simulink library "TestLib_BCM_Manager"  (Simulink 7.5)
settings: Solver=ode1  StartTime=0.0  StopTime=Inf  FixedStep=0.001  RelTol=1e-3
PostLoadFcn:
  | , if any(exist('dsrtsu_mdlpostloadfcn', 'file') == [2, 3, 6]), try dsrtsu_mdlpostloadfcn('Execute', bdroot); catch fprintf('Error in PostLoadFcn (dsrtsu_mdlpostloadfcn) for model "%s":\n %s\n', bdroot, lasterr); end, end,
undefined symbols (not defined in the file): cal, tloop
libraries: simulink x92, EC2_libraries x74
(part 2 of 2)

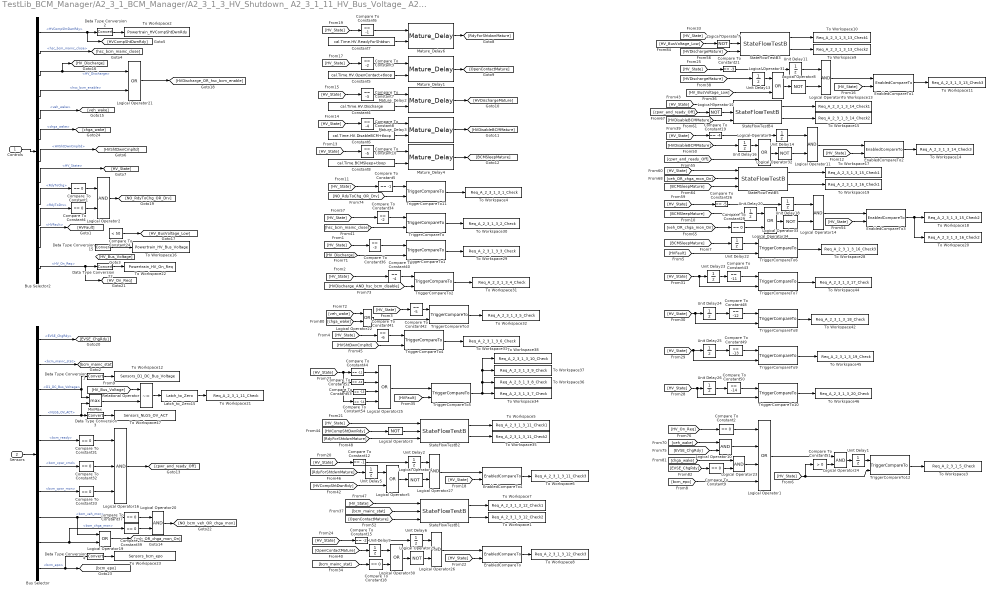
== system TestLib_BCM_Manager/A2_3_1_BCM_Manager/A2_3_1_3_HV_Shutdown_ A2_3_1_11_HV_Bus_Voltage_ A2_3_1_5_Startup_to_Shutdown ==
  Controls : Inport  OutDataType=fixdt(1, 16)  OutScaling=2^0
  Sensors : Inport  Port=2  OutDataType=fixdt(1, 16)  OutScaling=2^0
  Bus Selector : BusSelector  OutputSignals=Analog.EVSE_ChgRdy,Sensors_CAN.BCM_HS_Tx.BCM_Status.bcm_mainc_stat,Sensors_CAN.MCU_HS_Tx.M167_Voltage_Info.D1_DC_Bus_Voltage,Sensors_CAN.OBC_HS_Tx.NLG5_ACT_I.NLG5_OV_ACT,Sensors_CAN.BCM_HS_Tx.BCM_Status.bcm_ready,Sensors_CAN.BCM_HS_Tx.BCM_Status.bcm_cpwr_cmd,Sensors_CAN.BCM_HS_Tx.BCM_Status.bcm_cpwr_mon,Sensors_CAN.BCM_HS_Tx.BCM_Data1.bcm_veh_mon,Sensors_CAN.BCM_HS_Tx.BCM_Data1.bcm_chga_mon,Sensors_CAN.BCM_HS_Tx.BCM_Status.bcm_epo
  Bus Selector2 : BusSelector  OutputSignals=Powertrain_SC_Controls.HV_Status.HVCompShtDwnRdy,Powertrain_SC_Controls.BCM_Control.hsc_bcm_mainc_close,Powertrain_SC_Controls.HV_Status.HV_Discharge,Powertrain_SC_Controls.BCM_Control.hsc_bcm_enable,Powertrain_SC_Controls.BCM_Control.veh_wake,Powertrain_SC_Controls.BCM_Control.chga_wake,Powertrain_SC_Controls.HV_Status.HVShtDwnCmpltd,Powertrain_SC_Controls.HV_Status.HV_State,Powertrain_SC_Controls.HV_Status.RdyToChg,Powertrain_SC_Controls.HV_Status.RdyToDrv,Powertrain_SC_Controls.HV_Status.HVFault,Powertrain_SC_Controls.HV_Status.HV_On_Req
  Compare To Constant{1..2,4,9,18,29,31..33,37,39} (11 alike) : simulink/Logic and Bit Operations/Compare To Constant  SystemSampleTime=-1  relop===  const=0  LogicOutDataTypeMode=uint8
  Compare To Constant10 : simulink/Logic and Bit Operations/Compare To Constant  SystemSampleTime=-1  relop===  const=-5  LogicOutDataTypeMode=uint8
  Compare To Constant12 : simulink/Logic and Bit Operations/Compare To Constant  SystemSampleTime=-1  relop===  const=-1  LogicOutDataTypeMode=uint8
  Compare To Constant15 : simulink/Logic and Bit Operations/Compare To Constant  SystemSampleTime=-1  relop===  const=-2  LogicOutDataTypeMode=uint8
  Compare To Constant19 : simulink/Logic and Bit Operations/Compare To Constant  SystemSampleTime=-1  relop===  const=-4  LogicOutDataTypeMode=uint8
  Compare To Constant21 : simulink/Logic and Bit Operations/Compare To Constant  SystemSampleTime=-1  relop===  const=-3  LogicOutDataTypeMode=uint8
  Compare To Constant24 : simulink/Logic and Bit Operations/Compare To Constant  SystemSampleTime=-1  relop=<  const=50  LogicOutDataTypeMode=boolean
  Compare To Constant26 : simulink/Logic and Bit Operations/Compare To Constant  SystemSampleTime=-1  relop===  const=-5  LogicOutDataTypeMode=uint8
  Compare To Constant3 : simulink/Logic and Bit Operations/Compare To Constant  SystemSampleTime=-1  relop===  const=-2  LogicOutDataTypeMode=uint8
  Compare To Constant34 : simulink/Logic and Bit Operations/Compare To Constant  SystemSampleTime=-1  relop===  const=-2  LogicOutDataTypeMode=uint8
  Compare To Constant36 : simulink/Logic and Bit Operations/Compare To Constant  SystemSampleTime=-1  relop===  const=-3  LogicOutDataTypeMode=uint8
  Compare To Constant40 : simulink/Logic and Bit Operations/Compare To Constant  SystemSampleTime=-1  relop===  const=-4  LogicOutDataTypeMode=uint8
  Compare To Constant41 : simulink/Logic and Bit Operations/Compare To Constant  SystemSampleTime=-1  relop===  const=-6  LogicOutDataTypeMode=uint8
  Compare To Constant42 : simulink/Logic and Bit Operations/Compare To Constant  SystemSampleTime=-1  relop===  const=-5  LogicOutDataTypeMode=uint8
  Compare To Constant43 : simulink/Logic and Bit Operations/Compare To Constant  SystemSampleTime=-1  relop===  const=-11  LogicOutDataTypeMode=uint8
  Compare To Constant44 : simulink/Logic and Bit Operations/Compare To Constant  SystemSampleTime=-1  relop===  const=-11  LogicOutDataTypeMode=uint8
  Compare To Constant48 : simulink/Logic and Bit Operations/Compare To Constant  SystemSampleTime=-1  relop===  const=-12  LogicOutDataTypeMode=uint8
  Compare To Constant49 : simulink/Logic and Bit Operations/Compare To Constant  SystemSampleTime=-1  relop===  const=-13  LogicOutDataTypeMode=uint8
  Compare To Constant5 : simulink/Logic and Bit Operations/Compare To Constant  SystemSampleTime=-1  relop===  const=-1  LogicOutDataTypeMode=uint8
  Compare To Constant50 : simulink/Logic and Bit Operations/Compare To Constant  SystemSampleTime=-1  relop===  const=-14  LogicOutDataTypeMode=uint8
  Compare To Constant51 : simulink/Logic and Bit Operations/Compare To Constant  SystemSampleTime=-1  relop=>  const=0  LogicOutDataTypeMode=uint8
  Compare To Constant52 : simulink/Logic and Bit Operations/Compare To Constant  SystemSampleTime=-1  relop===  const=-12  LogicOutDataTypeMode=uint8
  Compare To Constant53 : simulink/Logic and Bit Operations/Compare To Constant  SystemSampleTime=-1  relop===  const=-13  LogicOutDataTypeMode=uint8
  Compare To Constant54 : simulink/Logic and Bit Operations/Compare To Constant  SystemSampleTime=-1  relop===  const=-14  LogicOutDataTypeMode=uint8
  Compare To Constant6 : simulink/Logic and Bit Operations/Compare To Constant  SystemSampleTime=-1  relop===  const=-1  LogicOutDataTypeMode=uint8
  Compare To Constant7 : simulink/Logic and Bit Operations/Compare To Constant  SystemSampleTime=-1  relop===  const=-3  LogicOutDataTypeMode=uint8
  Compare To Constant8 : simulink/Logic and Bit Operations/Compare To Constant  SystemSampleTime=-1  relop===  const=-4  LogicOutDataTypeMode=uint8
  Constant4 : Constant  Value=cal.Time.HV.Discharge  VectorParams1D=off
  Constant5 : Constant  Value=cal.Time.HV.OpenContact+tloop  VectorParams1D=off
  Constant6 : Constant  Value=cal.Time.HV.DisableBCM+tloop  VectorParams1D=off
  Constant7 : Constant  Value=cal.Time.HV.ReadyForShtdwn  VectorParams1D=off
  Constant8 : Constant  Value=cal.Time.BCMSleep+tloop  VectorParams1D=off
  Data Type Conversion{1..4,15,22} (6 alike) : DataTypeConversion  OutDataType=fixdt(1, 16)  OutScaling=2^0
  EnabledCompareTo : EC2_libraries/EnabledCompareTo  SystemSampleTime=-1  exp_val=-2
  EnabledCompareTo1 : EC2_libraries/EnabledCompareTo  SystemSampleTime=-1  exp_val=-3
  EnabledCompareTo2 : EC2_libraries/EnabledCompareTo  SystemSampleTime=-1  exp_val=-4
  EnabledCompareTo3 : EC2_libraries/EnabledCompareTo  SystemSampleTime=-1  exp_val=-5
  EnabledCompareTo4 : EC2_libraries/EnabledCompareTo  SystemSampleTime=-1  exp_val=-1
  Latch_to_Zero15 : EC2_libraries/Latch_to_Zero  SystemSampleTime=-1
  Logical Operator1 : Logic  Operator=OR  Inputs=4  AllPortsSameDT=off  OutDataTypeMode=boolean  OutDataTypeStr=boolean
  Logical Operator{2,6,10..11,14,20,23..24,26..27} (10 alike) : Logic  AllPortsSameDT=off  OutDataTypeMode=boolean  OutDataTypeStr=boolean
  Logical Operator{3..4,7..8,12,29,32..33} (8 alike) : Logic  Operator=NOT  AllPortsSameDT=off  OutDataTypeMode=boolean  OutDataTypeStr=boolean
  Logical Operator16 : Logic  Inputs=3  AllPortsSameDT=off  OutDataTypeMode=boolean  OutDataTypeStr=boolean
  Logical Operator{5,9,19,21..22,30..31,34} (8 alike) : Logic  Operator=OR  AllPortsSameDT=off  OutDataTypeMode=boolean  OutDataTypeStr=boolean
  Logical Operator25 : Logic  Operator=OR  Inputs=4  AllPortsSameDT=off  OutDataTypeMode=boolean  OutDataTypeStr=boolean
  Mature_Delay{1..4,6} (5 alike) : EC2_libraries/Mature_Delay  SystemSampleTime=-1
  MinMax : MinMax  Function=max  Inputs=2  OutDataType=fixdt(1, 16)  OutScaling=2^0
  Relational Operator : RelationalOperator  Operator=~=  LogicOutDataTypeMode=boolean  LogicDataType=fixdt(0, 8)  OutDataTypeStr=boolean
  StateFlowTestB1 : EC2_libraries/StateFlowTestB  SystemSampleTime=-1  StateBase=-2  PrimaryState=-3  SecondaryState=-12
  StateFlowTestB2 : EC2_libraries/StateFlowTestB  SystemSampleTime=-1  StateBase=-1  PrimaryState=-2  SecondaryState=-11
  StateFlowTestB3 : EC2_libraries/StateFlowTestB  SystemSampleTime=-1  StateBase=-3  PrimaryState=-4  SecondaryState=-13
  StateFlowTestB4 : EC2_libraries/StateFlowTestB  SystemSampleTime=-1  StateBase=-4  PrimaryState=-5  SecondaryState=-14
  StateFlowTestB5 : EC2_libraries/StateFlowTestB  SystemSampleTime=-1  StateBase=-5  PrimaryState=-6  SecondaryState=-6
  To Workspace1 : ToWorkspace  VariableName=Req_A_2_3_1_3_12_Check2  SampleTime=-1  SaveFormat=Array
      settings: Decimation=WORKSPACE_DECIMATION
  To Workspace10 : ToWorkspace  VariableName=Req_A_2_3_1_3_13_Check1  SampleTime=-1  SaveFormat=Array
      settings: Decimation=WORKSPACE_DECIMATION
  To Workspace11 : ToWorkspace  VariableName=Req_A_2_3_1_3_13_Check3  SampleTime=-1  SaveFormat=Array
      settings: Decimation=WORKSPACE_DECIMATION
  To Workspace12 : ToWorkspace  VariableName=Sensors_D1_DC_Bus_Voltage  SampleTime=-1  SaveFormat=Array
      settings: Decimation=WORKSPACE_DECIMATION
  To Workspace13 : ToWorkspace  VariableName=Req_A_2_3_1_3_14_Check1  SampleTime=-1  SaveFormat=Array
      settings: Decimation=WORKSPACE_DECIMATION
  To Workspace14 : ToWorkspace  VariableName=Req_A_2_3_1_3_14_Check3  SampleTime=-1  SaveFormat=Array
      settings: Decimation=WORKSPACE_DECIMATION
  To Workspace15 : ToWorkspace  VariableName=Req_A_2_3_1_3_14_Check2  SampleTime=-1  SaveFormat=Array
      settings: Decimation=WORKSPACE_DECIMATION
  To Workspace16 : ToWorkspace  VariableName=Powertrain_HV_Bus_Voltage  SampleTime=-1  SaveFormat=Array
      settings: Decimation=WORKSPACE_DECIMATION
  To Workspace17 : ToWorkspace  VariableName=Req_A_2_3_1_3_15_Check1  SampleTime=-1  SaveFormat=Array
      settings: Decimation=WORKSPACE_DECIMATION
  To Workspace18 : ToWorkspace  VariableName=Req_A_2_3_1_3_15_Check2  SampleTime=-1  SaveFormat=Array
      settings: Decimation=WORKSPACE_DECIMATION
  To Workspace19 : ToWorkspace  VariableName=Req_A_2_3_1_3_16_Check1  SampleTime=-1  SaveFormat=Array
      settings: Decimation=WORKSPACE_DECIMATION
  To Workspace2 : ToWorkspace  VariableName=Powertrain_HVCompShtDwnRdy  SampleTime=-1  SaveFormat=Array
      settings: Decimation=WORKSPACE_DECIMATION
  To Workspace20 : ToWorkspace  VariableName=Req_A_2_3_1_3_16_Check2  SampleTime=-1  SaveFormat=Array
      settings: Decimation=WORKSPACE_DECIMATION
  To Workspace21 : ToWorkspace  VariableName=Req_A_2_3_1_11_Check  SampleTime=-1  SaveFormat=Array
      settings: Decimation=WORKSPACE_DECIMATION
  To Workspace22 : ToWorkspace  VariableName=Powertrain_HV_On_Req  SampleTime=-1  SaveFormat=Array
      settings: Decimation=WORKSPACE_DECIMATION
  To Workspace23 : ToWorkspace  VariableName=Sensors_bcm_epo  SampleTime=-1  SaveFormat=Array
      settings: Decimation=WORKSPACE_DECIMATION
  To Workspace28 : ToWorkspace  VariableName=Req_A_2_3_1_3_16_Check3  SampleTime=-1  SaveFormat=Array
      settings: Decimation=WORKSPACE_DECIMATION
  To Workspace29 : ToWorkspace  VariableName=Req_A_2_3_1_3_3_Check  SampleTime=-1  SaveFormat=Array
      settings: Decimation=WORKSPACE_DECIMATION
  To Workspace3 : ToWorkspace  VariableName=Req_A_2_3_1_5_Check  SampleTime=-1  SaveFormat=Array
      settings: Decimation=WORKSPACE_DECIMATION
  To Workspace30 : ToWorkspace  VariableName=Req_A_2_3_1_3_2_Check  SampleTime=-1  SaveFormat=Array
      settings: Decimation=WORKSPACE_DECIMATION
  To Workspace31 : ToWorkspace  VariableName=Req_A_2_3_1_3_4_Check  SampleTime=-1  SaveFormat=Array
      settings: Decimation=WORKSPACE_DECIMATION
  To Workspace32 : ToWorkspace  VariableName=Req_A_2_3_1_3_5_Check  SampleTime=-1  SaveFormat=Array
      settings: Decimation=WORKSPACE_DECIMATION
  To Workspace33 : ToWorkspace  VariableName=Req_A_2_3_1_3_6_Check  SampleTime=-1  SaveFormat=Array
      settings: Decimation=WORKSPACE_DECIMATION
  To Workspace34 : ToWorkspace  VariableName=Req_A_2_3_1_3_7_Check  SampleTime=-1  SaveFormat=Array
      settings: Decimation=WORKSPACE_DECIMATION
  To Workspace35 : ToWorkspace  VariableName=Req_A_2_3_1_3_11_Check2  SampleTime=-1  SaveFormat=Array
      settings: Decimation=WORKSPACE_DECIMATION
  To Workspace36 : ToWorkspace  VariableName=Req_A_2_3_1_3_8_Check  SampleTime=-1  SaveFormat=Array
      settings: Decimation=WORKSPACE_DECIMATION
  To Workspace37 : ToWorkspace  VariableName=Req_A_2_3_1_3_9_Check  SampleTime=-1  SaveFormat=Array
      settings: Decimation=WORKSPACE_DECIMATION
  To Workspace38 : ToWorkspace  VariableName=Req_A_2_3_1_3_10_Check  SampleTime=-1  SaveFormat=Array
      settings: Decimation=WORKSPACE_DECIMATION
  To Workspace4 : ToWorkspace  VariableName=Req_A_2_3_1_3_1_Check  SampleTime=-1  SaveFormat=Array
      settings: Decimation=WORKSPACE_DECIMATION
  To Workspace42 : ToWorkspace  VariableName=Req_A_2_3_1_3_18_Check  SampleTime=-1  SaveFormat=Array
      settings: Decimation=WORKSPACE_DECIMATION
  To Workspace44 : ToWorkspace  VariableName=Req_A_2_3_1_3_17_Check  SampleTime=-1  SaveFormat=Array
      settings: Decimation=WORKSPACE_DECIMATION
  To Workspace45 : ToWorkspace  VariableName=Req_A_2_3_1_3_19_Check  SampleTime=-1  SaveFormat=Array
      settings: Decimation=WORKSPACE_DECIMATION
  To Workspace46 : ToWorkspace  VariableName=Req_A_2_3_1_3_20_Check  SampleTime=-1  SaveFormat=Array
      settings: Decimation=WORKSPACE_DECIMATION
  To Workspace47 : ToWorkspace  VariableName=Sensors_NLG5_OV_ACT  SampleTime=-1  SaveFormat=Array
      settings: Decimation=WORKSPACE_DECIMATION
  To Workspace5 : ToWorkspace  VariableName=Req_A_2_3_1_3_11_Check1  SampleTime=-1  SaveFormat=Array
      settings: Decimation=WORKSPACE_DECIMATION
  To Workspace6 : ToWorkspace  VariableName=Req_A_2_3_1_3_11_Check3  SampleTime=-1  SaveFormat=Array
      settings: Decimation=WORKSPACE_DECIMATION
  To Workspace7 : ToWorkspace  VariableName=Req_A_2_3_1_3_12_Check1  SampleTime=-1  SaveFormat=Array
      settings: Decimation=WORKSPACE_DECIMATION
  To Workspace8 : ToWorkspace  VariableName=Req_A_2_3_1_3_12_Check3  SampleTime=-1  SaveFormat=Array
      settings: Decimation=WORKSPACE_DECIMATION
  To Workspace9 : ToWorkspace  VariableName=Req_A_2_3_1_3_13_Check2  SampleTime=-1  SaveFormat=Array
      settings: Decimation=WORKSPACE_DECIMATION
  TriggerCompareTo : EC2_libraries/TriggerCompareTo  SystemSampleTime=-1  exp_val=0
  TriggerCompareTo{1,4..6,11} (5 alike) : EC2_libraries/TriggerCompareTo  SystemSampleTime=-1  exp_val=1
  TriggerCompareTo10 : EC2_libraries/TriggerCompareTo  SystemSampleTime=-1  exp_val=-5
  TriggerCompareTo12 : EC2_libraries/TriggerCompareTo  SystemSampleTime=-1  exp_val=-1
  TriggerCompareTo2 : EC2_libraries/TriggerCompareTo  SystemSampleTime=-1  exp_val=0
  TriggerCompareTo3 : EC2_libraries/TriggerCompareTo  SystemSampleTime=-1  exp_val=0
  TriggerCompareTo7 : EC2_libraries/TriggerCompareTo  SystemSampleTime=-1  exp_val=-2
  TriggerCompareTo8 : EC2_libraries/TriggerCompareTo  SystemSampleTime=-1  exp_val=-3
  TriggerCompareTo9 : EC2_libraries/TriggerCompareTo  SystemSampleTime=-1  exp_val=-4
  Unit Delay{1..2,5..6,9,11,13..14,16,18,20,22..26} (16 alike) : UnitDelay  SampleTime=-1
  wires:
  Compare To Constant2/1 -> Logical Operator1/1
  Logical Operator10/1 -> Logical Operator1/2
  TriggerCompareTo12/1 -> To Workspace3/1
  [veh_wake] -> Logical Operator10/1
  [EVSE_ChgRdy] -> Logical Operator10/2
  [HV_On_Req] -> Compare To Constant2/1
  [chga_wake] -> Logical Operator23/1
  Logical Operator23/1 -> Logical Operator1/3
  [EVSE_ChgRdy] -> Compare To Constant9/1
  Compare To Constant9/1 -> Logical Operator23/2
  Logical Operator1/1 -> Logical Operator24/1
  Logical Operator24/1 -> Unit Delay1/1
  Compare To Constant51/1 -> Logical Operator24/2
  Unit Delay1/1 -> TriggerCompareTo12/1
  [HV_State] -> TriggerCompareTo12/2, Compare To Constant51/1
  Logical Operator12/1 -> StateFlowTestB4/2
  Logical Operator7/1 -> StateFlowTestB3/2
  Logical Operator3/1 -> StateFlowTestB2/2
  [BCMSleepMature] -> StateFlowTestB5/3
  [HV_State] -> StateFlowTestB5/1
  [HV_State] -> StateFlowTestB4/1
  [cpwr_and_ready_Off] -> Logical Operator12/1
  [HV_BusVoltage_Low] -> Logical Operator7/1
  [HVCompShtDwnRdy] -> Logical Operator3/1
  [bcm_mainc_stat] -> StateFlowTestB1/2
  TriggerCompareTo11/1 -> To Workspace4/1
  Data Type Conversion3/1 -> To Workspace47/1
  Data Type Conversion1/1 -> To Workspace12/1
  Bus Selector/4 -> Data Type Conversion3/1, MinMax/2  "<NLG5_OV_ACT>"
  Bus Selector/3 -> Data Type Conversion1/1, MinMax/1  "<D1_DC_Bus_Voltage>"
  Compare To Constant50/1 -> TriggerCompareTo10/1
  Compare To Constant49/1 -> TriggerCompareTo9/1
  Compare To Constant48/1 -> TriggerCompareTo8/1
  Compare To Constant43/1 -> TriggerCompareTo7/1
  TriggerCompareTo10/1 -> To Workspace46/1
  TriggerCompareTo9/1 -> To Workspace45/1
  TriggerCompareTo7/1 -> To Workspace44/1
  TriggerCompareTo8/1 -> To Workspace42/1
  StateFlowTestB2/2 -> To Workspace35/1
  TriggerCompareTo5/1 -> To Workspace34/1, To Workspace36/1, To Workspace37/1, To Workspace38/1
  Compare To Constant41/1 -> TriggerCompareTo4/1
  Compare To Constant42/1 -> TriggerCompareTo3/1
  Compare To Constant40/1 -> TriggerCompareTo2/1
  Compare To Constant36/1 -> TriggerCompareTo1/1
  Compare To Constant34/1 -> TriggerCompareTo/1
  TriggerCompareTo4/1 -> To Workspace33/1
  TriggerCompareTo3/1 -> To Workspace32/1
  TriggerCompareTo2/1 -> To Workspace31/1
  TriggerCompareTo1/1 -> To Workspace29/1
  TriggerCompareTo/1 -> To Workspace30/1
  Bus Selector2/11 -> [HVFault]  "<HVFault>"
  Bus Selector2/6 -> [chga_wake]  "<chga_wake>"
  Bus Selector2/4 -> Logical Operator21/2  "<hsc_bcm_enable>"
  Bus Selector2/3 -> [HV_Discharge], Logical Operator21/1  "<HV_Discharge>"
  Controls/1 -> Bus Selector2/1
  Bus Selector2/5 -> [veh_wake]  "<veh_wake>"
  Bus Selector2/12 -> Data Type Conversion22/1, [HV_On_Req]  "<HV_On_Req>"
  TriggerCompareTo6/1 -> To Workspace28/1
  Compare To Constant39/1 -> Logical Operator20/2
  Compare To Constant37/1 -> Logical Operator20/1
  Compare To Constant33/1 -> Logical Operator16/3
  Compare To Constant32/1 -> Logical Operator16/2
  Compare To Constant31/1 -> Logical Operator16/1
  Bus Selector/9 -> Compare To Constant39/1, Logical Operator19/2  "<bcm_chga_mon>"
  Bus Selector/8 -> Logical Operator19/1, Compare To Constant37/1  "<bcm_veh_mon>"
  Bus Selector/7 -> Compare To Constant33/1  "<bcm_cpwr_mon>"
  Bus Selector/6 -> Compare To Constant32/1  "<bcm_cpwr_cmd>"
  Bus Selector/5 -> Compare To Constant31/1  "<bcm_ready>"
  Logical Operator5/1 -> Logical Operator4/1
  EnabledCompareTo4/1 -> To Workspace6/1
  StateFlowTestB2/1 -> To Workspace5/1
  Constant8/1 -> Mature_Delay4/2
  Compare To Constant10/1 -> Mature_Delay4/1
  Constant6/1 -> Mature_Delay3/2
  Compare To Constant8/1 -> Mature_Delay3/1
  Constant4/1 -> Mature_Delay2/2
  Compare To Constant7/1 -> Mature_Delay2/1
  Constant5/1 -> Mature_Delay1/2
  Compare To Constant3/1 -> Mature_Delay1/1
  Constant7/1 -> Mature_Delay6/2
  Compare To Constant6/1 -> Mature_Delay6/1
  Bus Selector2/1 -> Data Type Conversion2/1, [HVCompShtDwnRdy]  "<HVCompShtDwnRdy>"
  Data Type Conversion2/1 -> To Workspace2/1
  Bus Selector2/10 -> Compare To Constant4/1  "<RdyToDrv>"
  Bus Selector2/9 -> Compare To Constant1/1  "<RdyToChg>"
  Compare To Constant5/1 -> TriggerCompareTo11/1
  Compare To Constant4/1 -> Logical Operator2/2
  Compare To Constant1/1 -> Logical Operator2/1
  Bus Selector2/8 -> [HV_State]  "<HV_State>"
  Data Type Conversion22/1 -> To Workspace22/1
  Data Type Conversion15/1 -> To Workspace16/1
  Bus Selector/1 -> [EVSE_ChgRdy]  "<EVSE_ChgRdy>"
  Sensors/1 -> Bus Selector/1
  [HV_State] -> Compare To Constant34/1
  [HV_State] -> Compare To Constant36/1
  [HV_State] -> Compare To Constant40/1
  [HV_State] -> Compare To Constant42/1
  [HV_State] -> Compare To Constant41/1
  [HVFault] -> TriggerCompareTo6/2
  [HV_State] -> Compare To Constant5/1
  [HV_State] -> Compare To Constant3/1
  [HV_State] -> Compare To Constant7/1
  [HV_State] -> Compare To Constant8/1
  [HV_State] -> Compare To Constant10/1
  [HV_State] -> EnabledCompareTo4/2
  [HV_State] -> Compare To Constant6/1
  [HV_State] -> TriggerCompareTo10/2, Unit Delay26/1
  [HV_State] -> TriggerCompareTo7/2, Unit Delay23/1
  [HV_State] -> TriggerCompareTo8/2, Unit Delay24/1
  [HV_State] -> TriggerCompareTo9/2, Unit Delay25/1
  [HV_State] -> Compare To Constant44/1, Compare To Constant52/1, Compare To Constant53/1, Compare To Constant54/1
  [HVFault] -> TriggerCompareTo5/2
  Bus Selector/2 -> [bcm_mainc_stat]  "<bcm_mainc_stat>"
  [hsc_bcm_mainc_close] -> TriggerCompareTo/2
  Bus Selector2/2 -> [hsc_bcm_mainc_close]  "<hsc_bcm_mainc_close>"
  [HVCompShtDwnRdy] -> Logical Operator5/2
  [HVShtDwnCmpltd] -> TriggerCompareTo4/2
  Bus Selector2/7 -> [HVShtDwnCmpltd]  "<HVShtDwnCmpltd>"
  [RdyForShtdwnMature] -> StateFlowTestB2/3
  [RdyForShtdwnMature] -> Unit Delay5/1
  Mature_Delay6/1 -> [RdyForShtdwnMature]
  Mature_Delay1/1 -> [OpenContactMature]
  Mature_Delay2/1 -> [HVDischargeMature]
  Mature_Delay3/1 -> [HVDisableBCMMature]
  Mature_Delay4/1 -> [BCMSleepMature]
  Logical Operator16/1 -> [cpwr_and_ready_Off]
  Logical Operator19/1 -> [veh_OR_chga_mon_On]
  [HV_Discharge] -> TriggerCompareTo1/2
  Logical Operator22/1 -> TriggerCompareTo3/2
  [HVDischarge_AND_hsc_bcm_disable] -> TriggerCompareTo2/2
  Logical Operator21/1 -> [HVDischarge_OR_hsc_bcm_enable]
  Logical Operator2/1 -> [NO_RdyToChg_OR_Drv]
  [NO_RdyToChg_OR_Drv] -> TriggerCompareTo11/2
  Logical Operator20/1 -> [NO_bcm_veh_OR_chga_mon]
  MinMax/1 -> Relational Operator/2
  [veh_wake] -> Logical Operator22/1
  [chga_wake] -> Logical Operator22/2
  Compare To Constant24/1 -> [HV_BusVoltage_Low]
  Compare To Constant44/1 -> Logical Operator25/1
  Compare To Constant52/1 -> Logical Operator25/2
  Compare To Constant53/1 -> Logical Operator25/3
  Compare To Constant54/1 -> Logical Operator25/4
  Logical Operator25/1 -> TriggerCompareTo5/1
  Logical Operator4/1 -> Logical Operator27/2
  Logical Operator27/1 -> EnabledCompareTo4/1
  Compare To Constant12/1 -> Unit Delay2/1
  [HV_State] -> Compare To Constant12/1
  [HV_State] -> StateFlowTestB2/1
  Unit Delay2/1 -> Logical Operator27/1
  Unit Delay5/1 -> Logical Operator5/1
  StateFlowTestB1/2 -> To Workspace1/1
  Logical Operator30/1 -> Logical Operator29/1
  EnabledCompareTo/1 -> To Workspace8/1
  StateFlowTestB1/1 -> To Workspace7/1
  [HV_State] -> EnabledCompareTo/2
  [bcm_mainc_stat] -> Compare To Constant18/1
  [OpenContactMature] -> StateFlowTestB1/3
  [OpenContactMature] -> Unit Delay9/1
  [HV_State] -> StateFlowTestB1/1
  Logical Operator29/1 -> Logical Operator26/2
  Logical Operator26/1 -> EnabledCompareTo/1
  Compare To Constant15/1 -> Unit Delay6/1
  [HV_State] -> Compare To Constant15/1
  Unit Delay6/1 -> Logical Operator26/1
  Unit Delay9/1 -> Logical Operator30/1
  Compare To Constant18/1 -> Logical Operator30/2
  StateFlowTestB3/2 -> To Workspace9/1
  Logical Operator31/1 -> Logical Operator8/1
  EnabledCompareTo1/1 -> To Workspace11/1
  StateFlowTestB3/1 -> To Workspace10/1
  [HV_State] -> EnabledCompareTo1/2
  [HVDischargeMature] -> StateFlowTestB3/3
  [HVDischargeMature] -> Unit Delay13/1
  Logical Operator8/1 -> Logical Operator6/2
  Logical Operator6/1 -> EnabledCompareTo1/1
  Compare To Constant21/1 -> Unit Delay11/1
  [HV_State] -> Compare To Constant21/1
  [HV_State] -> StateFlowTestB3/1
  Unit Delay11/1 -> Logical Operator6/1
  Unit Delay13/1 -> Logical Operator31/1
  [HV_BusVoltage_Low] -> Logical Operator31/2
  StateFlowTestB4/2 -> To Workspace15/1
  Logical Operator9/1 -> Logical Operator32/1
  EnabledCompareTo2/1 -> To Workspace14/1
  StateFlowTestB4/1 -> To Workspace13/1
  [HV_State] -> EnabledCompareTo2/2
  [HVDisableBCMMature] -> StateFlowTestB4/3
  [HVDisableBCMMature] -> Unit Delay16/1
  Logical Operator32/1 -> Logical Operator11/2
  Logical Operator11/1 -> EnabledCompareTo2/1
  Compare To Constant19/1 -> Unit Delay14/1
  [HV_State] -> Compare To Constant19/1
  Unit Delay14/1 -> Logical Operator11/1
  Unit Delay16/1 -> Logical Operator9/1
  [cpwr_and_ready_Off] -> Logical Operator9/2
  Unit Delay22/1 -> TriggerCompareTo6/1
  StateFlowTestB5/2 -> To Workspace19/1
  Logical Operator34/1 -> Logical Operator33/1
  EnabledCompareTo3/1 -> To Workspace18/1, To Workspace20/1
  StateFlowTestB5/1 -> To Workspace17/1
  [HV_State] -> EnabledCompareTo3/2
  [BCMSleepMature] -> Unit Delay20/1
  Logical Operator33/1 -> Logical Operator14/2
  Logical Operator14/1 -> EnabledCompareTo3/1
  Compare To Constant26/1 -> Unit Delay18/1
  [HV_State] -> Compare To Constant26/1
  [veh_OR_chga_mon_On] -> StateFlowTestB5/2
  Unit Delay18/1 -> Logical Operator14/1
  Unit Delay20/1 -> Logical Operator34/1
  Compare To Constant29/1 -> Logical Operator34/2
  [veh_OR_chga_mon_On] -> Compare To Constant29/1
  [BCMSleepMature] -> Unit Delay22/1
  Unit Delay23/1 -> Compare To Constant43/1
  Unit Delay24/1 -> Compare To Constant48/1
  Unit Delay25/1 -> Compare To Constant49/1
  Unit Delay26/1 -> Compare To Constant50/1
  Latch_to_Zero15/1 -> To Workspace21/1
  Relational Operator/1 -> Latch_to_Zero15/1
  [HV_Bus_Voltage] -> Relational Operator/1
  Bus Selector/10 -> [bcm_epo], Data Type Conversion4/1  "<bcm_epo>"
  Data Type Conversion4/1 -> To Workspace23/1
  [bcm_epo] -> Logical Operator1/4

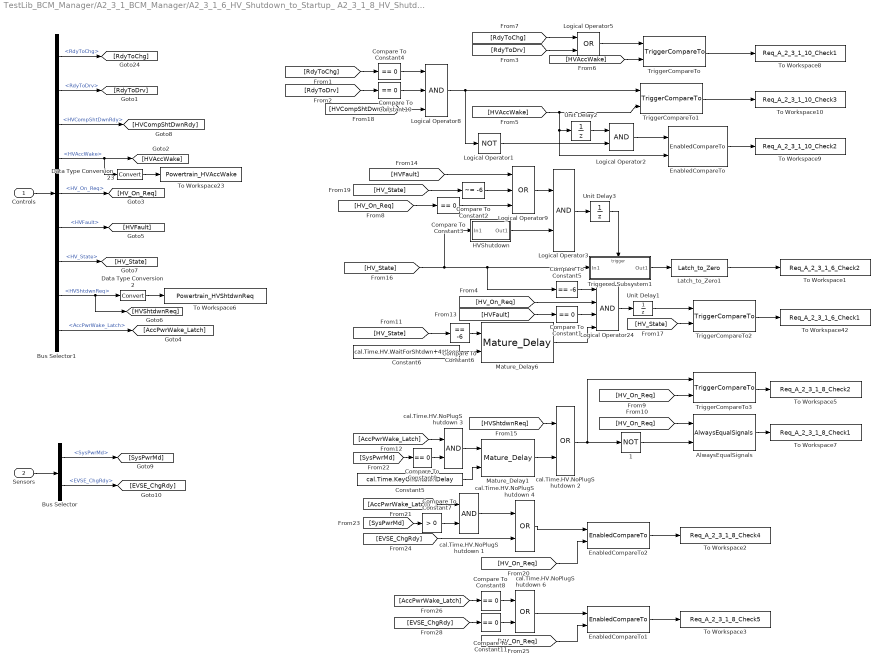
== system TestLib_BCM_Manager/A2_3_1_BCM_Manager/A2_3_1_6_HV_Shutdown_to_Startup_ A2_3_1_8_HV_Shutdown_Request_ A2_3_1_10_HV_Accessories_Wake_Up ==
  Controls : Inport  OutDataType=fixdt(1, 16)  OutScaling=2^0
  Sensors : Inport  Port=2  OutDataType=fixdt(1, 16)  OutScaling=2^0
  "  1" : Logic  Operator=NOT  AllPortsSameDT=off  OutDataTypeMode=boolean  OutDataTypeStr=boolean
  "      cal.Time.HV.NoPlugShutdown 1" : Logic  AllPortsSameDT=off  OutDataTypeMode=boolean  OutDataTypeStr=boolean
  "      cal.Time.HV.NoPlugShutdown 2" : Logic  Operator=OR  AllPortsSameDT=off  OutDataTypeMode=boolean  OutDataTypeStr=boolean
  "      cal.Time.HV.NoPlugShutdown 3" : Logic  AllPortsSameDT=off  OutDataTypeMode=boolean  OutDataTypeStr=boolean
  "      cal.Time.HV.NoPlugShutdown 4" : Logic  Operator=OR  AllPortsSameDT=off  OutDataTypeMode=boolean  OutDataTypeStr=boolean
  "      cal.Time.HV.NoPlugShutdown 6" : Logic  Operator=OR  AllPortsSameDT=off  OutDataTypeMode=boolean  OutDataTypeStr=boolean
  AlwaysEqualSignals : EC2_libraries/AlwaysEqualSignals  SystemSampleTime=-1
  Bus Selector : BusSelector  OutputSignals=Sensors_CAN.BodyCM_HS_Tx.PPEI_Platform_General_Status.SysPwrMd,Analog.EVSE_ChgRdy
  Bus Selector1 : BusSelector  OutputSignals=Powertrain_SC_Controls.HV_Status.RdyToChg,Powertrain_SC_Controls.HV_Status.RdyToDrv,Powertrain_SC_Controls.HV_Status.HVCompShtDwnRdy,Powertrain_SC_Controls.HV_Status.HVAccWake,Powertrain_SC_Controls.HV_Status.HV_On_Req,Powertrain_SC_Controls.HV_Status.HVFault,Powertrain_SC_Controls.HV_Status.HV_State,Powertrain_SC_Controls.HV_Status.HVShtdwnReq,Powertrain_SC_Controls.HV_Status.AccPwrWake_Latch
  Compare To Constant{1,3..4,10} (4 alike) : simulink/Logic and Bit Operations/Compare To Constant  SystemSampleTime=-1  relop===  const=0  LogicOutDataTypeMode=uint8
  Compare To Constant11 : simulink/Logic and Bit Operations/Compare To Constant  SystemSampleTime=-1  relop===  const=0  LogicOutDataTypeMode=boolean
  Compare To Constant2 : simulink/Logic and Bit Operations/Compare To Constant  SystemSampleTime=-1  relop=~=  const=-6  LogicOutDataTypeMode=uint8
  Compare To Constant5 : simulink/Logic and Bit Operations/Compare To Constant  SystemSampleTime=-1  relop===  const=-6  LogicOutDataTypeMode=uint8
  Compare To Constant6 : simulink/Logic and Bit Operations/Compare To Constant  SystemSampleTime=-1  relop===  const=-6  LogicOutDataTypeMode=uint8
  Compare To Constant7 : simulink/Logic and Bit Operations/Compare To Constant  SystemSampleTime=-1  relop=>  const=0  LogicOutDataTypeMode=boolean
  Compare To Constant8 : simulink/Logic and Bit Operations/Compare To Constant  SystemSampleTime=-1  relop===  const=0  LogicOutDataTypeMode=boolean
  Compare To Constant9 : simulink/Logic and Bit Operations/Compare To Constant  SystemSampleTime=-1  relop===  const=0  LogicOutDataTypeMode=boolean
  Constant5 : Constant  Value=cal.Time.KeyOffShtdwnDelay  VectorParams1D=off
  Constant6 : Constant  Value=cal.Time.HV.WaitForShtdwn+4*tloop  VectorParams1D=off
  Data Type Conversion2 : DataTypeConversion  OutDataType=fixdt(1, 16)  OutScaling=2^0
  Data Type Conversion23 : DataTypeConversion  OutDataType=fixdt(1, 16)  OutScaling=2^0
  EnabledCompareTo : EC2_libraries/EnabledCompareTo  SystemSampleTime=-1  exp_val=1
  EnabledCompareTo1 : EC2_libraries/EnabledCompareTo  SystemSampleTime=-1  exp_val=0
  EnabledCompareTo2 : EC2_libraries/EnabledCompareTo  SystemSampleTime=-1  exp_val=1
  HVShutdown : Subsystem  TreatAsAtomicUnit=on
  Latch_to_Zero1 : EC2_libraries/Latch_to_Zero  SystemSampleTime=-1
  Logical Operator1 : Logic  Operator=NOT  Inputs=3  AllPortsSameDT=off  OutDataTypeMode=boolean  OutDataTypeStr=boolean
  Logical Operator2 : Logic  AllPortsSameDT=off  OutDataTypeMode=boolean  OutDataTypeStr=boolean
  Logical Operator24 : Logic  Inputs=4  AllPortsSameDT=off  OutDataTypeMode=boolean  OutDataTypeStr=boolean
  Logical Operator3 : Logic  AllPortsSameDT=off  OutDataTypeMode=boolean  OutDataTypeStr=boolean
  Logical Operator5 : Logic  Operator=OR  AllPortsSameDT=off  OutDataTypeMode=boolean  OutDataTypeStr=boolean
  Logical Operator8 : Logic  Inputs=3  AllPortsSameDT=off  OutDataTypeMode=boolean  OutDataTypeStr=boolean
  Logical Operator9 : Logic  Operator=OR  Inputs=3  AllPortsSameDT=off  OutDataTypeMode=boolean  OutDataTypeStr=boolean
  Mature_Delay1 : EC2_libraries/Mature_Delay  SystemSampleTime=-1
  Mature_Delay6 : EC2_libraries/Mature_Delay  SystemSampleTime=-1
  To Workspace1 : ToWorkspace  VariableName=Req_A_2_3_1_6_Check2  SampleTime=-1  SaveFormat=Array
      settings: Decimation=WORKSPACE_DECIMATION
  To Workspace10 : ToWorkspace  VariableName=Req_A_2_3_1_10_Check3  SampleTime=-1  SaveFormat=Array
      settings: Decimation=WORKSPACE_DECIMATION
  To Workspace2 : ToWorkspace  VariableName=Req_A_2_3_1_8_Check4  SampleTime=-1  SaveFormat=Array
      settings: Decimation=WORKSPACE_DECIMATION
  To Workspace23 : ToWorkspace  VariableName=Powertrain_HVAccWake  SampleTime=-1  SaveFormat=Array
      settings: Decimation=WORKSPACE_DECIMATION
  To Workspace3 : ToWorkspace  VariableName=Req_A_2_3_1_8_Check5  SampleTime=-1  SaveFormat=Array
      settings: Decimation=WORKSPACE_DECIMATION
  To Workspace42 : ToWorkspace  VariableName=Req_A_2_3_1_6_Check1  SampleTime=-1  SaveFormat=Array
      settings: Decimation=WORKSPACE_DECIMATION
  To Workspace5 : ToWorkspace  VariableName=Req_A_2_3_1_8_Check2  SampleTime=-1  SaveFormat=Array
      settings: Decimation=WORKSPACE_DECIMATION
  To Workspace6 : ToWorkspace  VariableName=Powertrain_HVShtdwnReq  SampleTime=-1  SaveFormat=Array
      settings: Decimation=WORKSPACE_DECIMATION
  To Workspace7 : ToWorkspace  VariableName=Req_A_2_3_1_8_Check1  SampleTime=-1  SaveFormat=Array
      settings: Decimation=WORKSPACE_DECIMATION
  To Workspace8 : ToWorkspace  VariableName=Req_A_2_3_1_10_Check1  SampleTime=-1  SaveFormat=Array
      settings: Decimation=WORKSPACE_DECIMATION
  To Workspace9 : ToWorkspace  VariableName=Req_A_2_3_1_10_Check2  SampleTime=-1  SaveFormat=Array
      settings: Decimation=WORKSPACE_DECIMATION
  TriggerCompareTo : EC2_libraries/TriggerCompareTo  SystemSampleTime=-1  exp_val=1
  TriggerCompareTo1 : EC2_libraries/TriggerCompareTo  SystemSampleTime=-1  exp_val=0
  TriggerCompareTo2 : EC2_libraries/TriggerCompareTo  SystemSampleTime=-1  exp_val=1
  TriggerCompareTo3 : EC2_libraries/TriggerCompareTo  SystemSampleTime=-1  exp_val=0
  Triggered Subsystem1 : Subsystem  TreatAsAtomicUnit=on
  Unit Delay1 : UnitDelay  SampleTime=-1
  Unit Delay2 : UnitDelay  SampleTime=-1
  Unit Delay3 : UnitDelay  SampleTime=-1
  wires:
  Compare To Constant11/1 -> "      cal.Time.HV.NoPlugShutdown 6"/2
  Compare To Constant8/1 -> "      cal.Time.HV.NoPlugShutdown 6"/1
  EnabledCompareTo1/1 -> To Workspace3/1
  "      cal.Time.HV.NoPlugShutdown 6"/1 -> EnabledCompareTo1/1
  [EVSE_ChgRdy] -> Compare To Constant11/1
  [AccPwrWake_Latch] -> Compare To Constant8/1
  [HV_On_Req] -> EnabledCompareTo1/2
  EnabledCompareTo2/1 -> To Workspace2/1
  "      cal.Time.HV.NoPlugShutdown 4"/1 -> EnabledCompareTo2/1
  [EVSE_ChgRdy] -> "      cal.Time.HV.NoPlugShutdown 4"/2
  "      cal.Time.HV.NoPlugShutdown 1"/1 -> "      cal.Time.HV.NoPlugShutdown 4"/1
  Bus Selector/2 -> [EVSE_ChgRdy]  "<EVSE_ChgRdy>"
  Compare To Constant7/1 -> "      cal.Time.HV.NoPlugShutdown 1"/2
  [AccPwrWake_Latch] -> "      cal.Time.HV.NoPlugShutdown 1"/1
  [SysPwrMd] -> Compare To Constant7/1
  [SysPwrMd] -> Compare To Constant9/1
  [HV_On_Req] -> EnabledCompareTo2/2
  [AccPwrWake_Latch] -> "      cal.Time.HV.NoPlugShutdown 3"/1
  Compare To Constant9/1 -> "      cal.Time.HV.NoPlugShutdown 3"/2
  Bus Selector1/9 -> [AccPwrWake_Latch]  "<AccPwrWake_Latch>"
  Logical Operator8/1 -> TriggerCompareTo1/1, Logical Operator1/1
  TriggerCompareTo1/1 -> To Workspace10/1
  EnabledCompareTo/1 -> To Workspace9/1
  TriggerCompareTo/1 -> To Workspace8/1
  Bus Selector1/4 -> Data Type Conversion23/1, [HVAccWake]  "<HVAccWake>"
  "  1"/1 -> AlwaysEqualSignals/2
  AlwaysEqualSignals/1 -> To Workspace7/1
  "      cal.Time.HV.NoPlugShutdown 2"/1 -> TriggerCompareTo3/1, "  1"/1
  Mature_Delay1/1 -> "      cal.Time.HV.NoPlugShutdown 2"/2
  Bus Selector1/8 -> Data Type Conversion2/1, [HVShtdwnReq]  "<HVShtdwnReq>"
  Data Type Conversion2/1 -> To Workspace6/1
  Bus Selector/1 -> [SysPwrMd]  "<SysPwrMd>"
  Constant5/1 -> Mature_Delay1/2
  "      cal.Time.HV.NoPlugShutdown 3"/1 -> Mature_Delay1/1
  TriggerCompareTo3/1 -> To Workspace5/1
  Latch_to_Zero1/1 -> To Workspace1/1
  Triggered Subsystem1/1(Out1) -> Latch_to_Zero1/1
  Logical Operator24/1 -> Unit Delay1/1
  Compare To Constant1/1 -> Logical Operator24/3
  TriggerCompareTo2/1 -> To Workspace42/1
  Sensors/1 -> Bus Selector/1
  Controls/1 -> Bus Selector1/1
  Data Type Conversion23/1 -> To Workspace23/1
  [RdyToChg] -> Compare To Constant4/1
  [RdyToChg] -> Logical Operator5/1
  Bus Selector1/1 -> [RdyToChg]  "<RdyToChg>"
  [RdyToDrv] -> Logical Operator5/2
  [RdyToDrv] -> Compare To Constant10/1
  Bus Selector1/2 -> [RdyToDrv]  "<RdyToDrv>"
  [HVAccWake] -> TriggerCompareTo/2
  [HVAccWake] -> TriggerCompareTo1/2, EnabledCompareTo/2, Unit Delay2/1
  Logical Operator5/1 -> TriggerCompareTo/1
  Compare To Constant10/1 -> Logical Operator8/2
  Compare To Constant4/1 -> Logical Operator8/1
  Unit Delay2/1 -> Logical Operator2/1
  Logical Operator1/1 -> Logical Operator2/2
  Logical Operator2/1 -> EnabledCompareTo/1
  [HV_On_Req] -> AlwaysEqualSignals/1
  [HV_On_Req] -> TriggerCompareTo3/2
  [HV_On_Req] -> Compare To Constant3/1
  [HV_On_Req] -> Logical Operator24/2
  Bus Selector1/5 -> [HV_On_Req]  "<HV_On_Req>"
  [HVFault] -> Logical Operator9/1
  Bus Selector1/6 -> [HVFault]  "<HVFault>"
  [HVFault] -> Compare To Constant1/1
  [HVShtdwnReq] -> "      cal.Time.HV.NoPlugShutdown 2"/1
  [HV_State] -> Triggered Subsystem1/1(In1), Compare To Constant5/1, HVShutdown/1(In1)
  [HV_State] -> TriggerCompareTo2/2
  Bus Selector1/7 -> [HV_State]  "<HV_State>"
  [HVCompShtDwnRdy] -> Logical Operator8/3
  Bus Selector1/3 -> [HVCompShtDwnRdy]  "<HVCompShtDwnRdy>"
  Compare To Constant5/1 -> Logical Operator24/1
  Unit Delay1/1 -> TriggerCompareTo2/1
  Logical Operator9/1 -> Logical Operator3/1
  Logical Operator3/1 -> Unit Delay3/1
  HVShutdown/1(Out1) -> Logical Operator3/2
  Compare To Constant3/1 -> Logical Operator9/3
  Compare To Constant2/1 -> Logical Operator9/2
  [HV_State] -> Compare To Constant2/1
  Unit Delay3/1 -> Triggered Subsystem1/Trigger
  Constant6/1 -> Mature_Delay6/2
  Compare To Constant6/1 -> Mature_Delay6/1
  [HV_State] -> Compare To Constant6/1
  Mature_Delay6/1 -> Logical Operator24/4

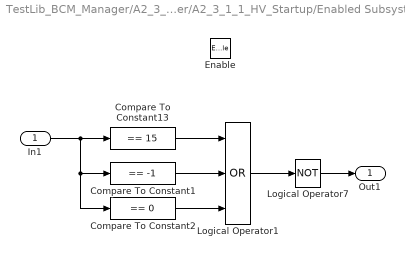
== system TestLib_BCM_Manager/A2_3_1_BCM_Manager/A2_3_1_1_HV_Startup/Enabled Subsystem ==
  In1 : Inport  OutDataType=fixdt(1, 16)  OutScaling=2^0
  Enable : EnablePort
  Compare To Constant1 : simulink/Logic and Bit Operations/Compare To Constant  SystemSampleTime=-1  relop===  const=-1  LogicOutDataTypeMode=boolean
  Compare To Constant13 : simulink/Logic and Bit Operations/Compare To Constant  SystemSampleTime=-1  relop===  const=15  LogicOutDataTypeMode=boolean
  Compare To Constant2 : simulink/Logic and Bit Operations/Compare To Constant  SystemSampleTime=-1  relop===  const=0  LogicOutDataTypeMode=boolean
  Logical Operator1 : Logic  Operator=OR  Inputs=3  AllPortsSameDT=off  OutDataTypeMode=boolean  OutDataTypeStr=boolean
  Logical Operator7 : Logic  Operator=NOT  AllPortsSameDT=off  OutDataTypeMode=boolean  OutDataTypeStr=boolean
  Out1 : Outport  OutDataType=fixdt(1, 16)  OutScaling=2^0
  wires:
  In1/1 -> Compare To Constant2/1, Compare To Constant1/1, Compare To Constant13/1
  Logical Operator1/1 -> Logical Operator7/1
  Compare To Constant2/1 -> Logical Operator1/3
  Compare To Constant1/1 -> Logical Operator1/2
  Compare To Constant13/1 -> Logical Operator1/1
  Logical Operator7/1 -> Out1/1

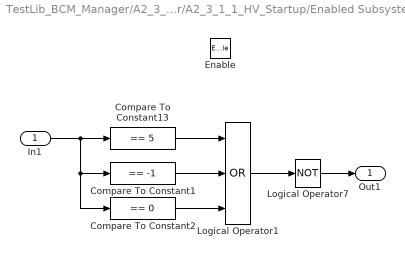
== system TestLib_BCM_Manager/A2_3_1_BCM_Manager/A2_3_1_1_HV_Startup/Enabled Subsystem1 ==
  In1 : Inport  OutDataType=fixdt(1, 16)  OutScaling=2^0
  Enable : EnablePort
  Compare To Constant1 : simulink/Logic and Bit Operations/Compare To Constant  SystemSampleTime=-1  relop===  const=-1  LogicOutDataTypeMode=boolean
  Compare To Constant13 : simulink/Logic and Bit Operations/Compare To Constant  SystemSampleTime=-1  relop===  const=5  LogicOutDataTypeMode=boolean
  Compare To Constant2 : simulink/Logic and Bit Operations/Compare To Constant  SystemSampleTime=-1  relop===  const=0  LogicOutDataTypeMode=boolean
  Logical Operator1 : Logic  Operator=OR  Inputs=3  AllPortsSameDT=off  OutDataTypeMode=boolean  OutDataTypeStr=boolean
  Logical Operator7 : Logic  Operator=NOT  AllPortsSameDT=off  OutDataTypeMode=boolean  OutDataTypeStr=boolean
  Out1 : Outport  OutDataType=fixdt(1, 16)  OutScaling=2^0
  wires:
  In1/1 -> Compare To Constant2/1, Compare To Constant1/1, Compare To Constant13/1
  Logical Operator1/1 -> Logical Operator7/1
  Compare To Constant2/1 -> Logical Operator1/3
  Compare To Constant1/1 -> Logical Operator1/2
  Compare To Constant13/1 -> Logical Operator1/1
  Logical Operator7/1 -> Out1/1

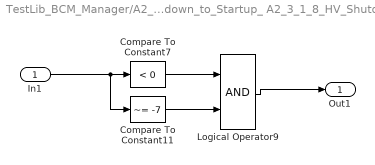
== system TestLib_BCM_Manager/A2_3_1_BCM_Manager/A2_3_1_6_HV_Shutdown_to_Startup_ A2_3_1_8_HV_Shutdown_Request_ A2_3_1_10_HV_Accessories_Wake_Up/HVShutdown ==
  In1 : Inport  OutDataType=fixdt(1, 16)  OutScaling=2^0
  Compare To Constant11 : simulink/Logic and Bit Operations/Compare To Constant  SystemSampleTime=-1  relop=~=  const=-7  LogicOutDataTypeMode=uint8
  Compare To Constant7 : simulink/Logic and Bit Operations/Compare To Constant  SystemSampleTime=-1  relop=<  const=0  LogicOutDataTypeMode=uint8
  Logical Operator9 : Logic  AllPortsSameDT=off  OutDataTypeMode=boolean  OutDataTypeStr=boolean
  Out1 : Outport  OutDataType=fixdt(1, 16)  OutScaling=2^0
  wires:
  In1/1 -> Compare To Constant7/1, Compare To Constant11/1
  Compare To Constant11/1 -> Logical Operator9/2
  Compare To Constant7/1 -> Logical Operator9/1
  Logical Operator9/1 -> Out1/1

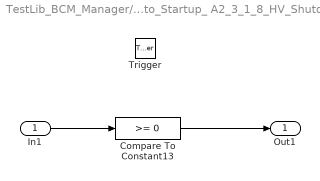
== system TestLib_BCM_Manager/A2_3_1_BCM_Manager/A2_3_1_6_HV_Shutdown_to_Startup_ A2_3_1_8_HV_Shutdown_Request_ A2_3_1_10_HV_Accessories_Wake_Up/Triggered Subsystem1 ==
  In1 : Inport  OutDataType=fixdt(1, 16)  OutScaling=2^0
  Trigger : TriggerPort
  Compare To Constant13 : simulink/Logic and Bit Operations/Compare To Constant  SystemSampleTime=-1  relop=>=  const=0  LogicOutDataTypeMode=boolean
  Out1 : Outport  OutDataType=fixdt(1, 16)  OutScaling=2^0
  wires:
  Compare To Constant13/1 -> Out1/1
  In1/1 -> Compare To Constant13/1
